simulink model "success"  (R2023b)
settings: Solver=ode45  StartTime=0.0  StopTime=2  RelTol=1e-3  EnableMultiTasking=on
libraries: spsSeriesRLCBranchLib x5, spsUniversalBridgeLib x5, spsThreePhaseSeriesRLCBranchLib x2, powerlib_extras x2, spsThreePhaseVIMeasurementLib x2, spsVoltageMeasurementLib x2, spsCurrentMeasurementLib x1, spsThreePhaseProgrammableVoltageSourceLib x1, dspfdesign x1, spsThreePhaseParallelRLCBranchLib x1, sps_lib x1, spsParallelRLCBranchLib x1
settings Model: Creator=vlc  LastModifiedBy=khana
settings SolverCC: AlgebraicLoopSolver=TrustRegion
settings DataIOCC: LimitDataPoints=on  SaveFormat=Array  SignalLoggingSaveFormat=ModelDataLogs  ReturnWorkspaceOutputs=off
settings OptimizationCC: ExpressionDepthLimit=2147483647  LifeSpan=inf
settings DebuggingCC: AlgebraicLoopMsg=none  UnderspecifiedInitializationDetection=Classic  MergeDetectMultiDrivingBlocksExec=none  FcnCallInpInsideContextMsg=warning  StateNameClashWarn=warning  SFUnexpectedBacktrackingDiag=warning  SFNoUnconditionalDefaultTransitionDiag=warning  SFExecutionAtInitializationDiag=none  ArithmeticOperatorsInVariantConditions=warning
settings HardwareCC: ProdBitPerPointer=32  ProdBitPerSizeT=32  ProdBitPerPtrDiffT=32  ProdLargestAtomicFloat=None  ProdIntDivRoundTo=Undefined  ProdEndianess=Unspecified  ProdWordSize=32  ProdHWDeviceType=32-bit Generic
settings ModelReferenceCC: PropagateSignalLabelsOutOfModel=off
settings SFSimCC: SimUseLocalCustomCode=off  CustomCodeUndefinedFunction=UseInterfaceOnly
settings RTWCC: RTWUseLocalCustomCode=off
settings CodeAppCC: StateflowObjectComments=on
settings GRTTargetCC: TargetLangStandard=C89/C90 (ANSI)  CombineOutputUpdateFcns=off  GRTInterface=on
settings ConfigComp: CovMetricSettings=dw  CovSaveCumulativeToWorkspaceVar=on  CovSaveSingleToWorkspaceVar=on  CovExternalEMLEnable=off
settings SimscapeCC: SimscapeNormalizeSystem=off

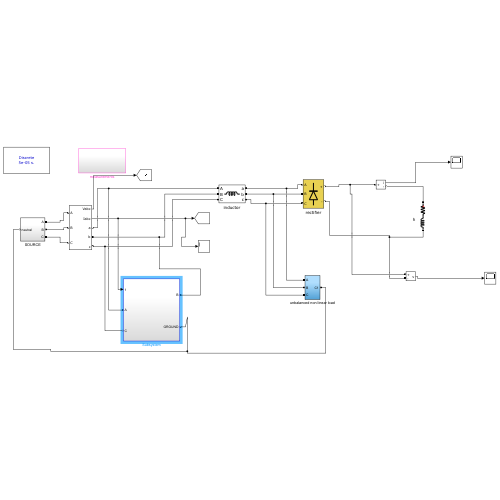
[thumbnail: Simulink's stored preview of the top-level diagram]
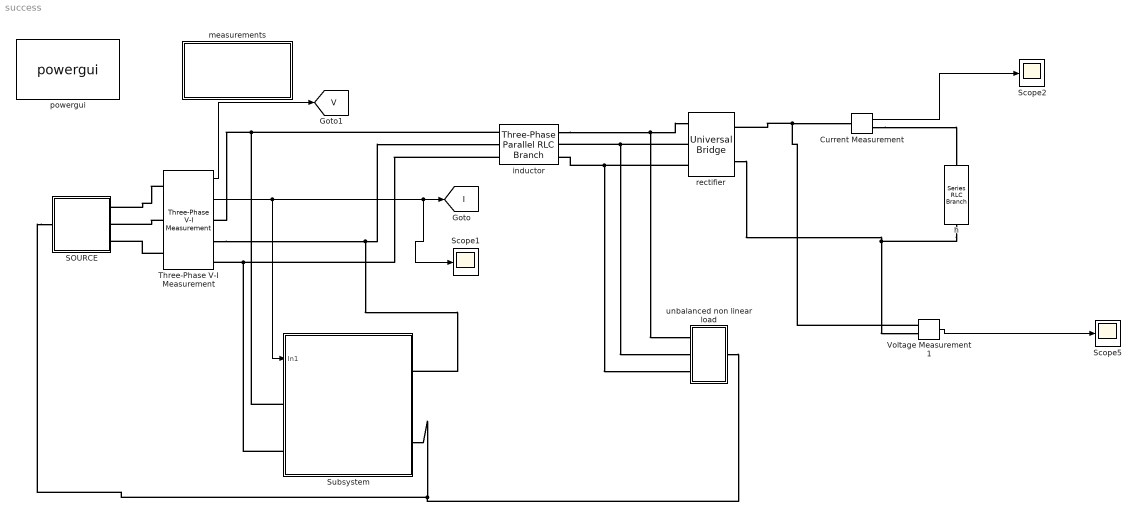
== system success ==
  " h" : spsSeriesRLCBranchLib/Series RLC Branch  LConnTagsString=__new0  RConnTagsString=__new0  BranchType=RL  Resistance=30  Inductance=.00030  SetiL0=off  InitialCurrent=0  Capacitance=1e-6  Setx0=off  InitialVoltage=0  Measurements=None
  Current Measurement : spsCurrentMeasurementLib/Current Measurement  PhasorSimulation=off  OutputType=Complex  PSBequivalent=0
  SOURCE : Subsystem
  Scope1 : Scope
  Scope2 : Scope
  Scope5 : Scope
  Subsystem : Subsystem
  Three-Phase V-I Measurement : spsThreePhaseVIMeasurementLib/Three-Phase V-I Measurement  VoltageMeasurement=phase-to-phase  SetLabelV=off  LabelV=Vabc  Vpu=off  VpuLL=off  CurrentMeasurement=yes  SetLabelI=off  LabelI=Iabc  Ipu=off  Pbase=100e6  Vbase=500e3  OutputType=Complex  PhasorSimulation=off  PSBequivalent=0
  Voltage Measurement1 : spsVoltageMeasurementLib/Voltage Measurement  PhasorSimulation=off  OutputType=Complex  PSBequivalent=0
  inductor : spsThreePhaseParallelRLCBranchLib/Three-Phase Parallel RLC Branch  LConnTagsString=A|B|C  RConnTagsString=A|B|C  BranchType=L  Resistance=1  Inductance=.0004  Capacitance=1e-6  Measurements=None
  measurements : Subsystem
  powergui : sps_lib/powergui  Priority=1  SimulationMode=Discrete  SampleTime=50e-6  frequency=60  Iterations=50  frequencyindice=0  Pbase=100e6  ErrMax=1e-4  UnitsV=kV  UnitsW=MW  buscounter=0  FunctionMessages=off  echomessages=off  EnableUseOfTLC=off  CurrentSourceSwitches=off  DisableSnubberDevices=off  DisableRonSwitches=off  DisableVfSwitches=off  DisplayEquations=off  AutomaticDiscreteSolvers=off  SolverType=Tustin/Backward Euler (TBE)  Interpol=off  ExternalGateDelay=off  methode=off  Ts=0  x0status=blocks  SPID=off  SwTol=0  HookPort=off  NonlinearTolerance=1e-4  nMaxIteration=100  ContinueOnMaxIteration=off  RestoreLinks=warning  ResistiveCurrentMeasurement=off  Frange=[0:2:500]  Ylog=off  Xlog=on  ShowGrid=off  save=off  variable=ZData  structure=Iabc  ZoomFFT=off  StartTime=0.05  cycles=10  DisplayStyle=1  fundamental=50  FreqAxis=on  MaxFrequency=1000  frequencyindicesteady=1  RmsSteady=1  display=off
  rectifier : spsUniversalBridgeLib/Universal Bridge  Arms=3  SnubberResistance=2000  SnubberCapacitance=0.1e-6  Device=Diodes  Ron=1e-3  Lon=0  ForwardVoltages="[  0  0  ]"  ForwardVoltage=0  GTOparameters=[ 10e-6 , 20e-6 ]  IGBTparameters=[ 1e-6 , 2e-6 ]  Measurements=None  Measurements_2=None  converterType=Rectifier
  unbalanced non linear load : Subsystem
  tag scope: I=global, V=global
  wires:
  Three-Phase V-I Measurement/2 -> [I], Scope1/1, Subsystem/1(In1)
  Three-Phase V-I Measurement/1 -> [V]
  Voltage Measurement1/1 -> Scope5/1
  Current Measurement/1 -> Scope2/1
  connections:
  Three-Phase V-I Measurement/LConn1 -- SOURCE/RConn1
  Three-Phase V-I Measurement/LConn3 -- SOURCE/RConn3
  Subsystem/LConn1 -- inductor/LConn1 -- Three-Phase V-I Measurement/RConn1
  Subsystem/RConn1 -- Three-Phase V-I Measurement/RConn2 -- inductor/LConn2
  Subsystem/LConn2 -- inductor/LConn3 -- Three-Phase V-I Measurement/RConn3
  Three-Phase V-I Measurement/LConn2 -- SOURCE/RConn2
  rectifier/LConn3 -- inductor/RConn3 -- unbalanced non linear load/LConn3
  rectifier/LConn2 -- inductor/RConn2 -- unbalanced non linear load/LConn2
  inductor/RConn1 -- rectifier/LConn1 -- unbalanced non linear load/LConn1
  Voltage Measurement1/LConn1 -- rectifier/RConn1 -- Current Measurement/LConn1
  " h"/RConn1 -- rectifier/RConn2 -- Voltage Measurement1/LConn2
  SOURCE/LConn1 -- unbalanced non linear load/RConn1 -- Subsystem/RConn2
  Current Measurement/RConn1 -- " h"/LConn1

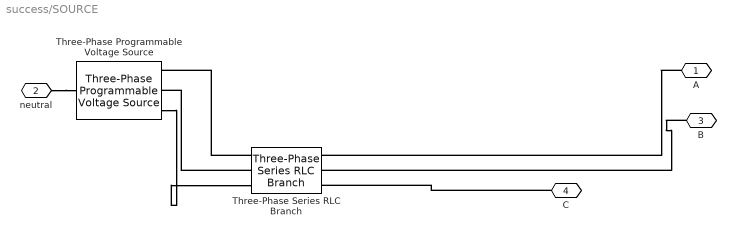
== system success/SOURCE ==
  Three-Phase Programmable Voltage Source : spsThreePhaseProgrammableVoltageSourceLib/Three-Phase Programmable Voltage Source  PositiveSequence=[220 0 50]  VariationEntity=None  VariationType=Step  VariationTypeAlt=Step  VariationStep=0.5  VariationRate=10  VariationMagnitude=0.3  VariationFrequency=2  VariationTiming=[1 2]  VariationPhaseA=off  Amplitudes=[1 0.8 1.2 1.0]  TimeValues=[0 0.1 0.15 0.2]  HarmonicGeneration=off  HarmonicA=[3 0.2 -25 0]  HarmonicB=[2 0.15 35 2]  Timing="[0.05  3]"  BusType=swing  Pref=0  Qref=0  Qmin=-inf  Qmax=inf
  Three-Phase Series RLC Branch : spsThreePhaseSeriesRLCBranchLib/Three-Phase Series RLC Branch  LConnTagsString=A|B|C  RConnTagsString=A|B|C  BranchType=L  Resistance=.01  Inductance=.000010  Capacitance=1e-6  Measurements=Branch voltages and currents
  A : PMIOPort  Side=Right
  neutral : PMIOPort  Port=2  Side=Left
  B : PMIOPort  Port=3  Side=Right
  C : PMIOPort  Port=4  Side=Right
  connections:
  Three-Phase Series RLC Branch/LConn1 -- Three-Phase Programmable Voltage Source/RConn1
  neutral/RConn1 -- Three-Phase Programmable Voltage Source/LConn1
  A/RConn1 -- Three-Phase Series RLC Branch/RConn1
  Three-Phase Series RLC Branch/LConn2 -- Three-Phase Programmable Voltage Source/RConn2
  Three-Phase Programmable Voltage Source/RConn3 -- Three-Phase Series RLC Branch/LConn3
  B/RConn1 -- Three-Phase Series RLC Branch/RConn2
  C/RConn1 -- Three-Phase Series RLC Branch/RConn3

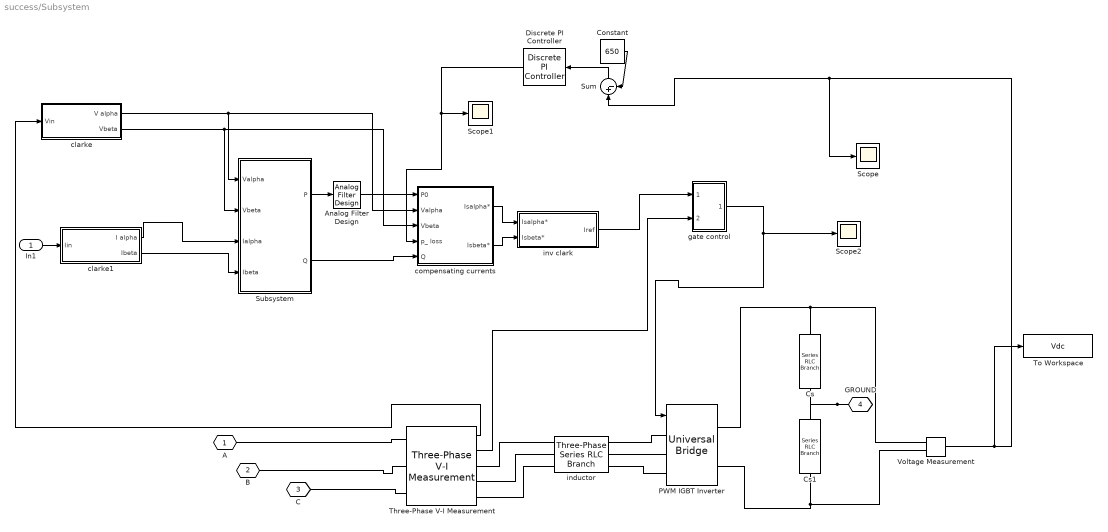
== system success/Subsystem ==
  In1 : Inport
  Analog Filter Design : dspfdesign/Analog Filter Design  method=Butterworth  filttype=Lowpass  N=8  Wlo=30  Whi=80  Rp=2  Rs=40
  Constant : Constant  Value=650
  Cs : spsSeriesRLCBranchLib/Series RLC Branch  LConnTagsString=__new0  RConnTagsString=__new0  BranchType=C  Resistance=1  Inductance=1e-3  SetiL0=off  InitialCurrent=0  Capacitance=.0000011  Setx0=off  InitialVoltage=0  Measurements=None
  Cs1 : spsSeriesRLCBranchLib/Series RLC Branch  LConnTagsString=__new0  RConnTagsString=__new0  BranchType=C  Resistance=1  Inductance=1e-3  SetiL0=off  InitialCurrent=0  Capacitance=.0000011  Setx0=off  InitialVoltage=0  Measurements=None
  Discrete PI Controller : powerlib_extras/Discrete  Control Blocks/Discrete PI Controller  Kp=0.1  Ki=1  Par_Limits=[1e6 -1e6]  Init=0  Ts=50e-6
  PWM IGBT Inverter : spsUniversalBridgeLib/Universal Bridge  Arms=3  SnubberResistance=5000  SnubberCapacitance=inf  Device=IGBT / Diodes  Ron=1e-3  Lon=0  ForwardVoltages="[  0.0  0.0  ]"  ForwardVoltage=.8  GTOparameters=[ 1e-6 ,1e-6 ]  IGBTparameters=[ 1e-6 , 5e-6 ]  Measurements=Device currents  Measurements_2=None  converterType=Rectifier
      settings: AttributesFormatString=\n
  Scope : Scope
  Scope1 : Scope
  Scope2 : Scope
  Subsystem : Subsystem
  Sum : Sum  Inputs=|+-
  Three-Phase V-I Measurement : spsThreePhaseVIMeasurementLib/Three-Phase V-I Measurement  VoltageMeasurement=phase-to-phase  SetLabelV=off  LabelV=Vabc  Vpu=off  VpuLL=off  CurrentMeasurement=yes  SetLabelI=off  LabelI=Iabc  Ipu=off  Pbase=100e6  Vbase=500e3  OutputType=Complex  PhasorSimulation=off  PSBequivalent=0
  To Workspace : ToWorkspace  VariableName=Vdc  SaveFormat=Timeseries  SampleTime=-1
  Voltage Measurement : spsVoltageMeasurementLib/Voltage Measurement  PhasorSimulation=off  OutputType=Complex  PSBequivalent=0
  clarke : Subsystem
  clarke1 : Subsystem
  compensating currents : Subsystem
  "gate control " : Subsystem
  inductor : spsThreePhaseSeriesRLCBranchLib/Three-Phase Series RLC Branch  LConnTagsString=A|B|C  RConnTagsString=A|B|C  BranchType=L  Resistance=1  Inductance=.0002  Capacitance=1e-6  Measurements=None
  inv clark : Subsystem
  A : PMIOPort  Tag=PMCPort  Side=Left
  B : PMIOPort  Tag=PMCPort  Port=2  Side=Right
  C : PMIOPort  Tag=PMCPort  Port=3  Side=Left
  GROUND : PMIOPort  Tag=PMCPort  Port=4  Side=Right
  wires:
  Voltage Measurement/1 -> To Workspace/1, Scope/1, Sum/1
  Constant/1 -> Sum/2
  Sum/1 -> Discrete PI Controller/1
  In1/1 -> clarke1/1(Iin)
  Subsystem/1(P) -> Analog Filter Design/1
  Discrete PI Controller/1 -> compensating currents/4(p_ loss), Scope1/1
  Analog Filter Design/1 -> compensating currents/1(P0)
  compensating currents/1(Isalpha*) -> inv clark/1(Isalpha*)
  compensating currents/2(Isbeta*) -> inv clark/2(Isbeta*)
  Three-Phase V-I Measurement/1 -> clarke/1(Vin)
  clarke/1(V alpha) -> Subsystem/1(Valpha), compensating currents/2(Valpha)
  clarke/2(Vbeta) -> Subsystem/2(Vbeta), compensating currents/3(Vbeta)
  clarke1/1(I alpha) -> Subsystem/3(Ialpha)
  inv clark/1(Iref) -> "gate control "/1(iref)
  Three-Phase V-I Measurement/2 -> "gate control "/2(imeas)
  "gate control "/1(Out1) -> PWM IGBT Inverter/1, Scope2/1
  clarke1/2(Ibeta) -> Subsystem/4(Ibeta)
  Subsystem/2(Q) -> compensating currents/5(Q)
  connections:
  Three-Phase V-I Measurement/LConn3 -- C/RConn1
  Three-Phase V-I Measurement/LConn2 -- B/RConn1
  Three-Phase V-I Measurement/RConn1 -- inductor/LConn1
  Voltage Measurement/LConn2 -- Cs1/RConn1 -- PWM IGBT Inverter/RConn2
  GROUND/RConn1 -- Cs/RConn1 -- Cs1/LConn1
  Voltage Measurement/LConn1 -- Cs/LConn1 -- PWM IGBT Inverter/RConn1
  Three-Phase V-I Measurement/LConn1 -- A/RConn1
  Three-Phase V-I Measurement/RConn2 -- inductor/LConn2
  Three-Phase V-I Measurement/RConn3 -- inductor/LConn3
  inductor/RConn1 -- PWM IGBT Inverter/LConn1
  inductor/RConn2 -- PWM IGBT Inverter/LConn2
  inductor/RConn3 -- PWM IGBT Inverter/LConn3

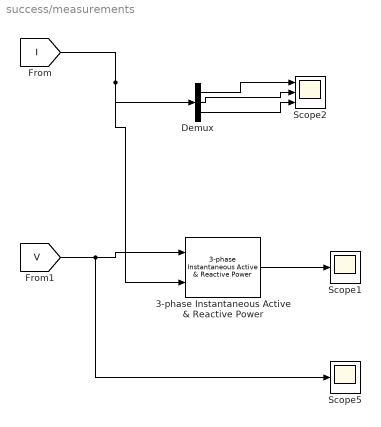
== system success/measurements ==
  3-phase Instantaneous Active & Reactive Power : powerlib_extras/Measurements/3-phase  Instantaneous  Active & Reactive Power
  Demux : Demux  Outputs=3
  Scope1 : Scope
  Scope2 : Scope  NumInputPorts=3
  Scope5 : Scope
  wires:
  [I] -> 3-phase Instantaneous Active & Reactive Power/2, Demux/1
  [V] -> 3-phase Instantaneous Active & Reactive Power/1, Scope5/1
  3-phase Instantaneous Active & Reactive Power/1 -> Scope1/1
  Demux/1 -> Scope2/1
  Demux/2 -> Scope2/2
  Demux/3 -> Scope2/3

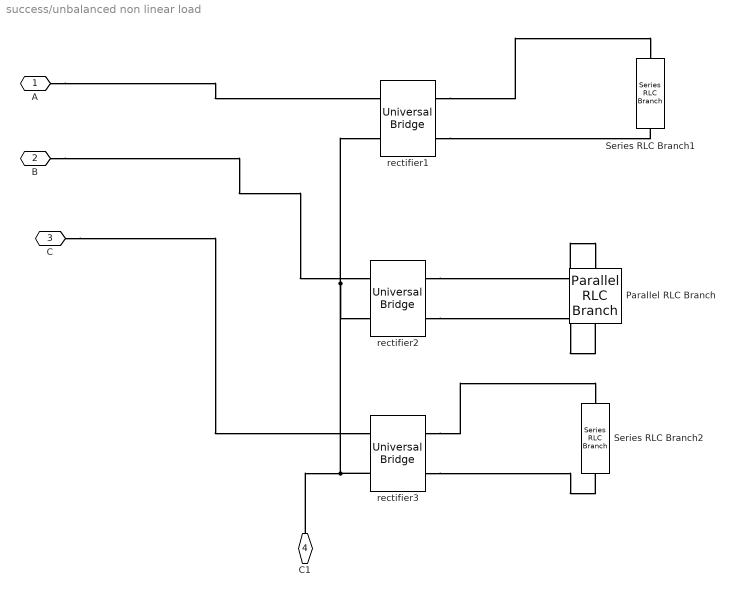
== system success/unbalanced non linear load ==
  Parallel RLC Branch : spsParallelRLCBranchLib/Parallel RLC Branch  LConnTagsString=a  RConnTagsString=__new0  BranchType=RC  Resistance=50  Inductance=1e-3  SetiL0=off  InitialCurrent=0  Capacitance=1e-6  Setx0=off  InitialVoltage=0  Measurements=None
  Series RLC Branch1 : spsSeriesRLCBranchLib/Series RLC Branch  LConnTagsString=__new0  RConnTagsString=__new0  BranchType=RL  Resistance=1e50  Inductance=.000100  SetiL0=off  InitialCurrent=0  Capacitance=1e-6  Setx0=off  InitialVoltage=0  Measurements=None
  Series RLC Branch2 : spsSeriesRLCBranchLib/Series RLC Branch  LConnTagsString=__new0  RConnTagsString=__new0  BranchType=R  Resistance=1  Inductance=1e-3  SetiL0=off  InitialCurrent=0  Capacitance=1e-6  Setx0=off  InitialVoltage=0  Measurements=None
  rectifier1 : spsUniversalBridgeLib/Universal Bridge  Arms=2  SnubberResistance=5000  SnubberCapacitance=inf  Device=Diodes  Ron=1e-3  Lon=0  ForwardVoltages="[  0  0  ]"  ForwardVoltage=0  GTOparameters=[ 10e-6 , 20e-6 ]  IGBTparameters=[ 1e-6 , 2e-6 ]  Measurements=None  Measurements_2=None  converterType=Rectifier
  rectifier2 : spsUniversalBridgeLib/Universal Bridge  Arms=2  SnubberResistance=5000  SnubberCapacitance=inf  Device=Diodes  Ron=1e-3  Lon=0  ForwardVoltages="[  0  0  ]"  ForwardVoltage=0  GTOparameters=[ 10e-6 , 20e-6 ]  IGBTparameters=[ 1e-6 , 2e-6 ]  Measurements=None  Measurements_2=None  converterType=Rectifier
  rectifier3 : spsUniversalBridgeLib/Universal Bridge  Arms=2  SnubberResistance=5000  SnubberCapacitance=inf  Device=Diodes  Ron=1e-3  Lon=0  ForwardVoltages="[  0  0  ]"  ForwardVoltage=0  GTOparameters=[ 10e-6 , 20e-6 ]  IGBTparameters=[ 1e-6 , 2e-6 ]  Measurements=None  Measurements_2=None  converterType=Rectifier
  A : PMIOPort  Side=Left
  B : PMIOPort  Port=2  Side=Left
  C : PMIOPort  Port=3  Side=Left
  C1 : PMIOPort  Port=4  Side=Right
  connections:
  B/RConn1 -- rectifier2/LConn1
  rectifier3/LConn2 -- rectifier1/LConn2 -- rectifier2/LConn2 -- C1/RConn1
  rectifier1/RConn1 -- Series RLC Branch1/LConn1
  rectifier1/RConn2 -- Series RLC Branch1/RConn1
  rectifier2/RConn1 -- Parallel RLC Branch/LConn1
  rectifier2/RConn2 -- Parallel RLC Branch/RConn1
  rectifier3/RConn1 -- Series RLC Branch2/LConn1
  rectifier3/RConn2 -- Series RLC Branch2/RConn1
  A/RConn1 -- rectifier1/LConn1
  C/RConn1 -- rectifier3/LConn1

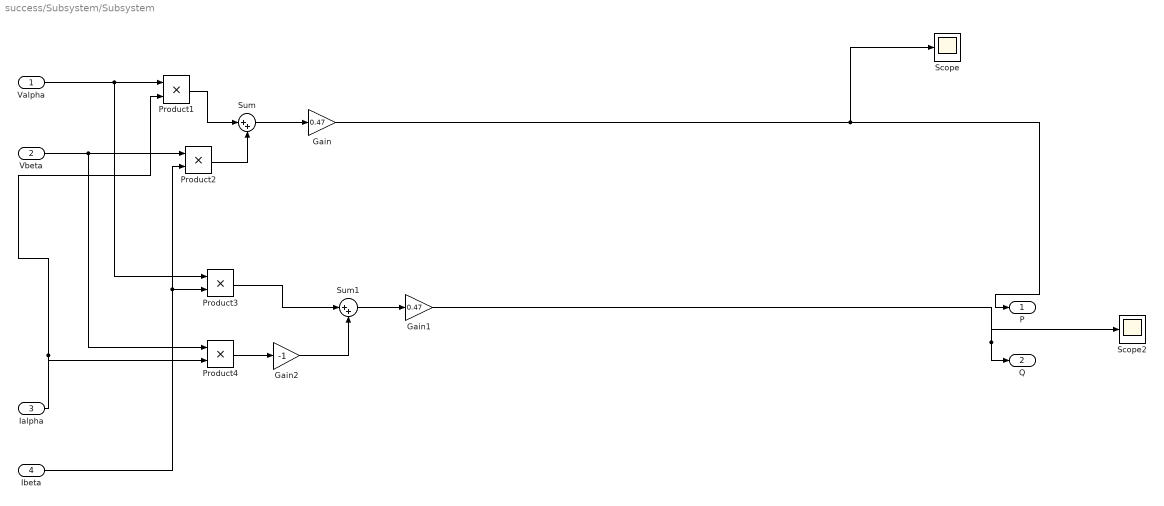
== system success/Subsystem/Subsystem ==
  Valpha : Inport
  Vbeta : Inport  Port=2
  Ialpha : Inport  Port=3
  Ibeta : Inport  Port=4
  Gain : Gain  Gain=0.47
  Gain1 : Gain  Gain=0.47
  Gain2 : Gain  Gain=-1
  Product{1..4} (4 alike) : Product  RndMeth=Zero
  Scope : Scope
  Scope2 : Scope
  Sum : Sum  Inputs=|++
  Sum1 : Sum  Inputs=|++
  P : Outport
  Q : Outport  Port=2
  wires:
  Ialpha/1 -> Product1/2, Product4/2
  Valpha/1 -> Product1/1, Product3/1
  Vbeta/1 -> Product2/1, Product4/1
  Ibeta/1 -> Product2/2, Product3/2
  Product1/1 -> Sum/1
  Product2/1 -> Sum/2
  Sum/1 -> Gain/1
  Gain/1 -> P/1, Scope/1
  Product4/1 -> Gain2/1
  Product3/1 -> Sum1/1
  Gain2/1 -> Sum1/2
  Sum1/1 -> Gain1/1
  Gain1/1 -> Q/1, Scope2/1

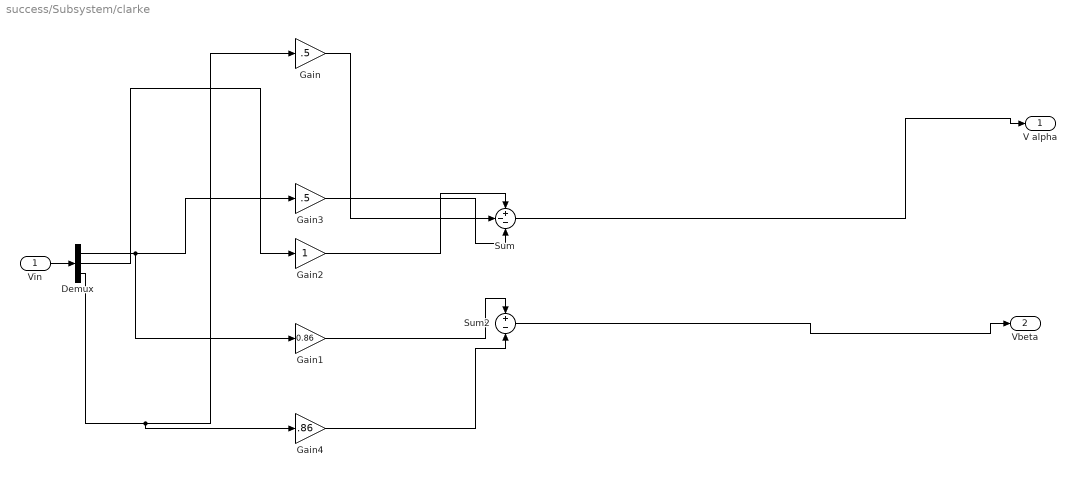
== system success/Subsystem/clarke ==
  Vin : Inport
  Demux : Demux  Outputs=3
  Gain : Gain  Gain=.5
  Gain1 : Gain  Gain=0.86
  Gain2 : Gain
  Gain3 : Gain  Gain=.5
  Gain4 : Gain  Gain=.86
  Sum : Sum  Inputs=+--
  Sum2 : Sum  Inputs=+-
  V alpha : Outport
  Vbeta : Outport  Port=2
  wires:
  Demux/2 -> Gain3/1, Gain1/1
  Demux/1 -> Gain2/1
  Demux/3 -> Gain/1, Gain4/1
  Gain2/1 -> Sum/1
  Gain/1 -> Sum/2
  Gain3/1 -> Sum/3
  Sum/1 -> V alpha/1
  Gain1/1 -> Sum2/1
  Gain4/1 -> Sum2/2
  Sum2/1 -> Vbeta/1
  Vin/1 -> Demux/1

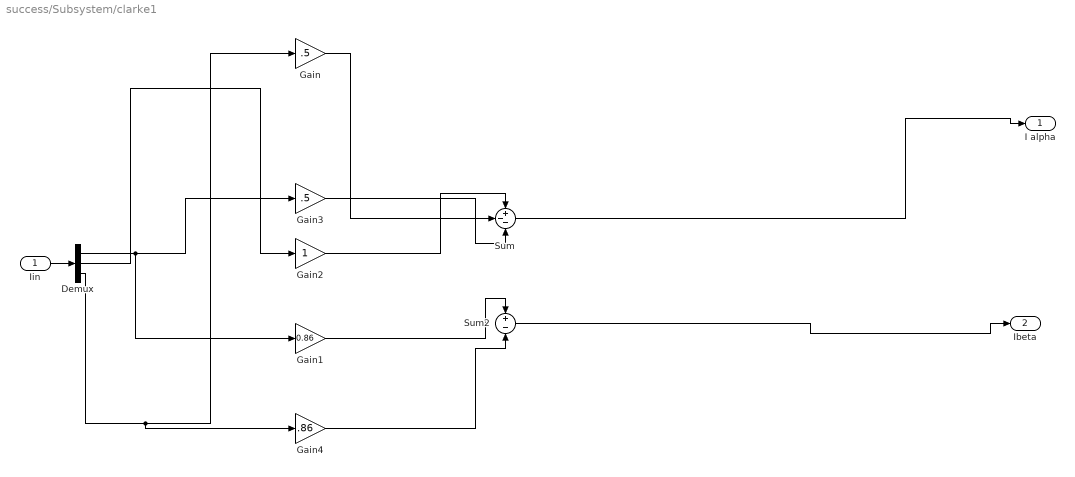
== system success/Subsystem/clarke1 ==
  Iin : Inport
  Demux : Demux  Outputs=3
  Gain : Gain  Gain=.5
  Gain1 : Gain  Gain=0.86
  Gain2 : Gain
  Gain3 : Gain  Gain=.5
  Gain4 : Gain  Gain=.86
  Sum : Sum  Inputs=+--
  Sum2 : Sum  Inputs=+-
  I alpha : Outport
  Ibeta : Outport  Port=2
  wires:
  Iin/1 -> Demux/1
  Sum2/1 -> Ibeta/1
  Gain4/1 -> Sum2/2
  Gain1/1 -> Sum2/1
  Sum/1 -> I alpha/1
  Gain3/1 -> Sum/3
  Gain/1 -> Sum/2
  Gain2/1 -> Sum/1
  Demux/3 -> Gain4/1, Gain/1
  Demux/1 -> Gain2/1
  Demux/2 -> Gain1/1, Gain3/1

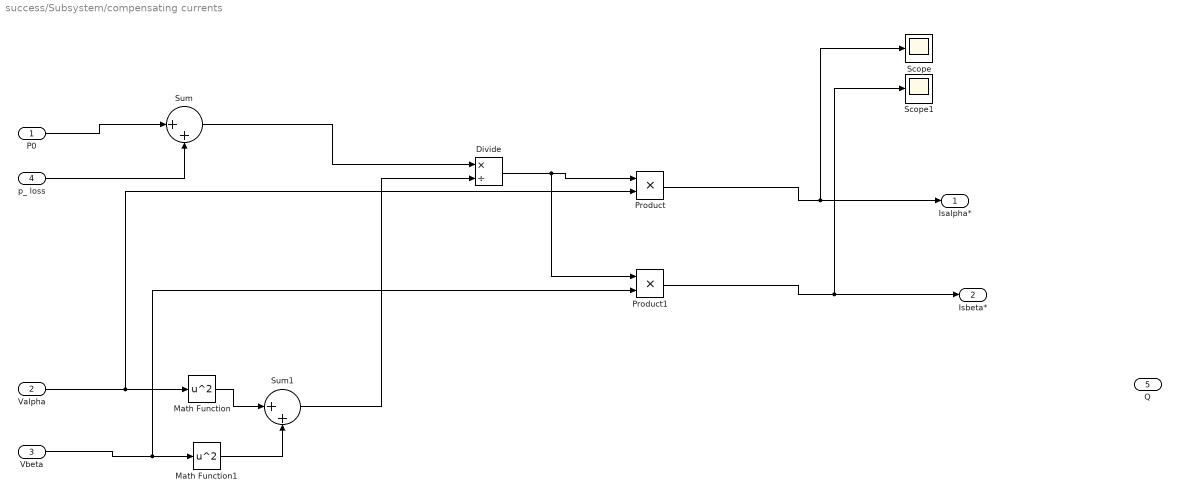
== system success/Subsystem/compensating currents ==
  P0 : Inport
  Valpha : Inport  Port=2
  Vbeta : Inport  Port=3
  p_ loss : Inport  Port=4
  Q : Inport  Port=5
  Divide : Product  Inputs=*/
  Math Function : Math  Operator=square  SignedPower=on
  Math Function1 : Math  Operator=square  SignedPower=on
  Product : Product  RndMeth=Zero
  Product1 : Product  RndMeth=Zero
  Scope : Scope
  Scope1 : Scope
  Sum : Sum  Inputs=|++
  Sum1 : Sum  Inputs=|++
  Isalpha* : Outport
  Isbeta* : Outport  Port=2
  wires:
  Valpha/1 -> Math Function/1, Product/2
  Vbeta/1 -> Math Function1/1, Product1/2
  Math Function/1 -> Sum1/1
  Math Function1/1 -> Sum1/2
  Sum/1 -> Divide/1
  Sum1/1 -> Divide/2
  Divide/1 -> Product/1, Product1/1
  Product1/1 -> Isbeta*/1, Scope1/1
  Product/1 -> Isalpha*/1, Scope/1
  P0/1 -> Sum/1
  p_ loss/1 -> Sum/2

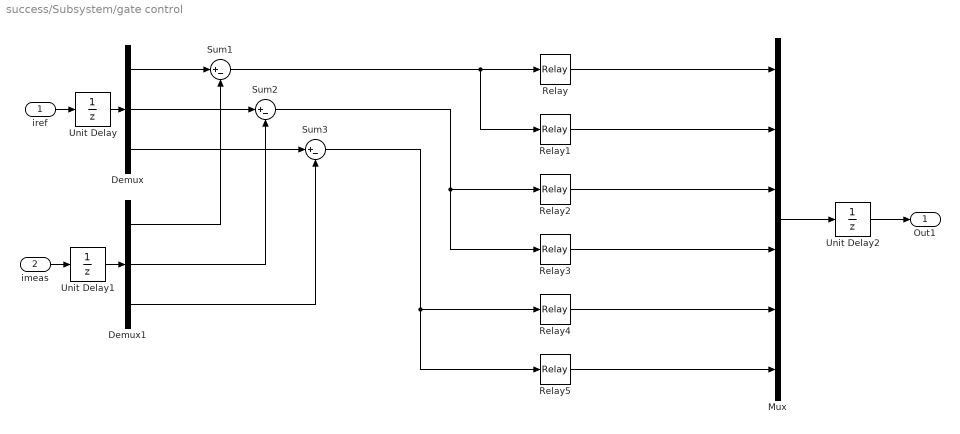
== system success/Subsystem/gate control  ==
  iref : Inport
  imeas : Inport  Port=2
  Demux : Demux  Outputs=3
  Demux1 : Demux  Outputs=3
  Mux : Mux  Inputs=6
  Relay : Relay
  Relay1 : Relay  OnOutputValue=0  OffOutputValue=1
  Relay2 : Relay
  Relay3 : Relay  OnOutputValue=0  OffOutputValue=1
  Relay4 : Relay
  Relay5 : Relay  OnOutputValue=0  OffOutputValue=1
  Sum1 : Sum  Inputs=|+-
  Sum2 : Sum  Inputs=|+-
  Sum3 : Sum  Inputs=|+-
  Unit Delay : UnitDelay  SampleTime=-1
  Unit Delay1 : UnitDelay  SampleTime=-1
  Unit Delay2 : UnitDelay  SampleTime=-1
  Out1 : Outport
  wires:
  Demux1/1 -> Sum1/2
  Demux1/2 -> Sum2/2
  Demux1/3 -> Sum3/2
  Demux/1 -> Sum1/1
  Demux/2 -> Sum2/1
  Demux/3 -> Sum3/1
  Sum1/1 -> Relay/1, Relay1/1
  Sum2/1 -> Relay2/1, Relay3/1
  Sum3/1 -> Relay5/1, Relay4/1
  Relay/1 -> Mux/1
  Relay1/1 -> Mux/2
  Relay2/1 -> Mux/3
  Relay3/1 -> Mux/4
  Relay4/1 -> Mux/5
  Relay5/1 -> Mux/6
  iref/1 -> Unit Delay/1
  Unit Delay/1 -> Demux/1
  imeas/1 -> Unit Delay1/1
  Unit Delay1/1 -> Demux1/1
  Mux/1 -> Unit Delay2/1
  Unit Delay2/1 -> Out1/1

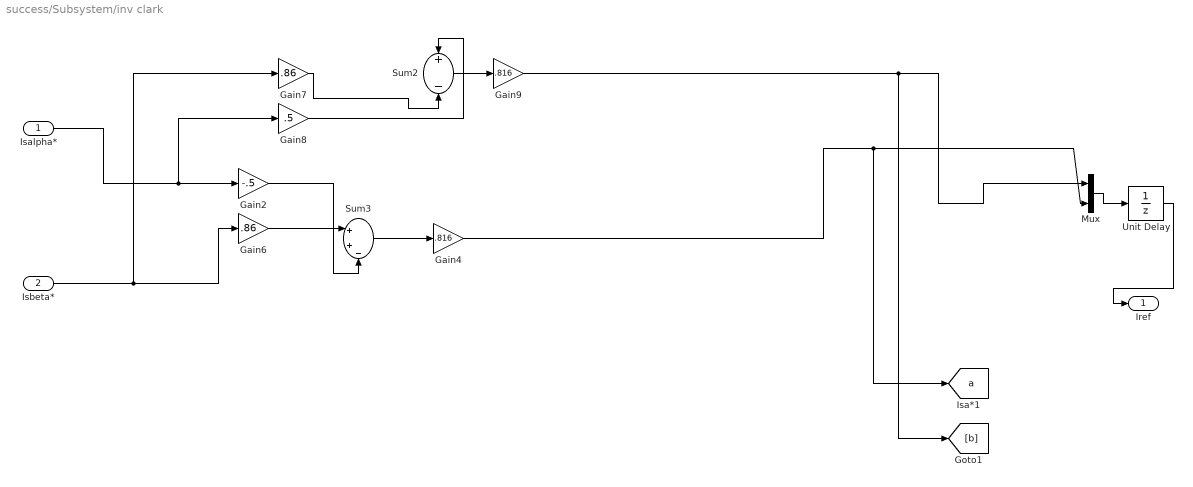
== system success/Subsystem/inv clark ==
  Isalpha* : Inport
  Isbeta* : Inport  Port=2
  Gain2 : Gain  Gain=-.5
  Gain4 : Gain  Gain=.816
  Gain6 : Gain  Gain=.86
  Gain7 : Gain  Gain=.86
  Gain8 : Gain  Gain=.5
  Gain9 : Gain  Gain=.816
  Mux : Mux  Inputs=2
  Sum2 : Sum  Inputs=+-
  Sum3 : Sum  Inputs=|++-
  Unit Delay : UnitDelay  SampleTime=-1
  Iref : Outport
  tag scope: a=global
  wires:
  Isalpha*/1 -> Gain2/1, Gain8/1
  Isbeta*/1 -> Gain6/1, Gain7/1
  Gain2/1 -> Sum3/3
  Gain6/1 -> Sum3/1
  Sum3/1 -> Gain4/1
  Gain7/1 -> Sum2/2
  Gain8/1 -> Sum2/1
  Sum2/1 -> Gain9/1
  Gain4/1 -> [a], Mux/2
  Gain9/1 -> [b], Mux/1
  Mux/1 -> Unit Delay/1
  Unit Delay/1 -> Iref/1
